simulink model "dbe_xaui_corr"  (Simulink 7.0)
settings: Solver=ode45  StartTime=0.0  StopTime=1000  RelTol=1e-3
undefined symbols (not defined in the file or in its folder): iBOB
libraries: xbsIndex_r4 x458, xps_library x38, casper_library_misc x12, casper_library_sources x2, gavrt_library x1, simulink x1, casper_library_scopes x1
(part 2 of 4)

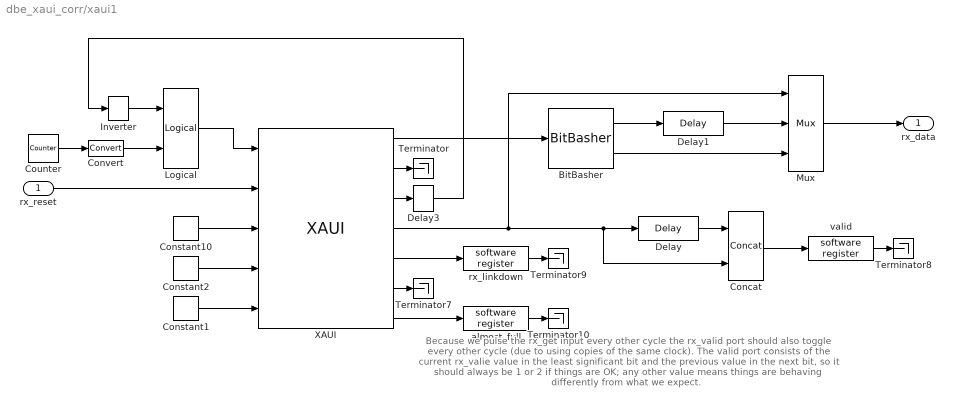
== system dbe_xaui_corr/xaui1 ==
  note: Because we pulse the rx_get input every other cycle
      | the rx_valid port should also toggle every other cycle
      | (due to using copies of the same clock).  The valid port
      | consists of the current rx_valie value in the least significant
      | bit and the previous value in the next bit, so it should
      | always be 1 or 2 if things are OK; any other value means
      | things are behaving differently from what we expect.
  rx_reset : Inport
  BitBasher : xbsIndex_r4/BitBasher  bitexpr=|  display_expr=off  sr_1=1  arith_type1=Unsigned  bin_pt1=0  sr_2=2  arith_type2=Unsigned  bin_pt2=0  sr_3=3  arith_type3=Unsigned  bin_pt3=0  sr_4=4  arith_type4=Unsigned  bin_pt4=0  dbl_ovrd=off  block_type=bitbasher
      | <html><head><meta name="qrichtext" content="1" /><style type="text/css">
      | p, li { white-space: pre-wrap; }
      | </style></head><body style=" font-family:'MS Shell Dlg 2'; font-size:8.25pt; font-weight:400; font-style:normal;">
      | <p style=" margin-top:12px; margin-bottom:12px; margin-left:0px; margin-right:0px; -qt-block-indent:0; text-indent:0px; font-family:'MS Shell Dlg'; font-size:8pt;">lo32={in64[31:0]}<br />hi32={in64[63:32]}</p></body></html>
      settings: block_version=10.1.3
  Concat : xbsIndex_r4/Concat  num_inputs=2  dbl_ovrd=off  block_type=concat
      settings: block_version=10.1.3
  Constant1 : xbsIndex_r4/Constant  arith_type=Boolean  const=0  n_bits=4  bin_pt=0  explicit_period=on  period=1  equ=P=C  opselect=C  inp2=PCIN>>17  opr=+  inp1=P  carry=CIN  dbl_ovrd=off  block_type=constant
      settings: block_version=11.3
  Constant10 : xbsIndex_r4/Constant  arith_type=Unsigned  const=2^4 -1  n_bits=32  bin_pt=0  explicit_period=on  period=1  equ=P=C  opselect=C  inp2=PCIN>>17  opr=+  inp1=P  carry=CIN  dbl_ovrd=off  block_type=constant
      settings: block_version=11.3
  Constant2 : xbsIndex_r4/Constant  arith_type=Unsigned  const=0  n_bits=4  bin_pt=0  explicit_period=on  period=1  equ=P=C  opselect=C  inp2=PCIN>>17  opr=+  inp1=P  carry=CIN  dbl_ovrd=off  block_type=constant
      settings: block_version=11.3
  Convert : xbsIndex_r4/Convert  arith_type=Boolean  n_bits=16  bin_pt=14  quantization=Truncate  overflow=Wrap  latency=0  dbl_ovrd=off  pipeline=off  block_type=convert
      settings: block_version=10.1.3
  Counter : xbsIndex_r4/Counter  cnt_type=Free Running  cnt_to=Inf  operation=Up  start_count=0  cnt_by_val=1  arith_type=Unsigned  n_bits=1  bin_pt=0  load_pin=off  rst=off  en=off  explicit_period=on  period=1  dbl_ovrd=off  use_behavioral_HDL=off  use_rpm=off  implementation=Fabric  block_type=counter
  Delay : xbsIndex_r4/Delay  en=off  latency=1  dbl_ovrd=off  reg_retiming=off  block_type=delay
  Delay1 : xbsIndex_r4/Delay  en=off  latency=1  dbl_ovrd=off  reg_retiming=off  block_type=delay
  Delay3 : xbsIndex_r4/Delay  en=off  latency=32  dbl_ovrd=off  reg_retiming=off  block_type=delay
      settings: block_version=11.3
  Inverter : xbsIndex_r4/Inverter  en=off  latency=0  dbl_ovrd=off  block_type=inv
      settings: block_version=11.3
  Logical : xbsIndex_r4/Logical  logical_function=AND  inputs=2  en=off  latency=0  precision=Full  arith_type=Unsigned  n_bits=16  bin_pt=0  align_bp=on  dbl_ovrd=off  block_type=logical
  Mux : xbsIndex_r4/Mux  inputs=2  en=off  latency=0  precision=Full  arith_type=Unsigned  n_bits=16  bin_pt=14  quantization=Truncate  overflow=Wrap  dbl_ovrd=off  block_type=mux
  Terminator{,7..10} (5 alike) : Terminator
  XAUI : xps_library/XAUI  Tag=xps:xaui  SystemSampleTime=-1  demux=1  port=iBOB:0  open_phy=off  show_param=off  pre_emph=3  swing=800
      link override convert_tx_data: n_bits=32
      link override convert_tx_outofband: n_bits=4
      link override dbe_xaui_corr_xaui1_XAUI_rx_data: n_bits=64
      link override dbe_xaui_corr_xaui1_XAUI_rx_outofband: n_bits=8
      link override dbe_xaui_corr_xaui_summer_XAUI0_rx_data: n_bits=32
      link override dbe_xaui_corr_xaui_summer_XAUI0_rx_outofband: n_bits=4
      link override dbe_xaui_xaui_summer_XAUI0_rx_data: n_bits=32
      link override dbe_xaui_xaui_summer_XAUI0_rx_outofband: n_bits=4
      link override xaui_XAUI_RECV_rx_data: n_bits=32
      link override xaui_XAUI_RECV_rx_outofband: n_bits=4
  almost_full : xps_library/software register  Tag=xps:sw_reg  SystemSampleTime=-1  io_dir=To Processor  arith_type=Unsigned  bitwidth=32  bin_pt=0  sample_period=1  gw_name=dbe_xaui_corr_xaui1_almost_full_user_data_in
      link override convert: arith_type=Unsigned  n_bits=32  bin_pt=0
  rx_linkdown : xps_library/software register  Tag=xps:sw_reg  SystemSampleTime=-1  io_dir=To Processor  arith_type=Unsigned  bitwidth=32  bin_pt=0  sample_period=1  gw_name=dbe_xaui_corr_xaui1_rx_linkdown_user_data_in
      link override convert: arith_type=Unsigned  n_bits=32  bin_pt=0
  valid : xps_library/software register  Tag=xps:sw_reg  SystemSampleTime=-1  io_dir=To Processor  arith_type=Unsigned  bitwidth=32  bin_pt=0  sample_period=1  gw_name=dbe_xaui_corr_xaui1_valid_user_data_in
      link override convert: arith_type=Unsigned  n_bits=32  bin_pt=0
  rx_data : Outport
  wires:
  XAUI/2 -> Terminator/1
  Constant2/1 -> XAUI/4
  XAUI/3 -> Delay3/1
  Delay3/1 -> Inverter/1
  XAUI/6 -> Terminator7/1
  Constant10/1 -> XAUI/3
  XAUI/4 -> Mux/1, Delay/1, Concat/2
  XAUI/5 -> rx_linkdown/1
  valid/1 -> Terminator8/1
  rx_linkdown/1 -> Terminator9/1
  almost_full/1 -> Terminator10/1
  XAUI/7 -> almost_full/1
  Constant1/1 -> XAUI/5
  rx_reset/1 -> XAUI/2
  Inverter/1 -> Logical/1
  Logical/1 -> XAUI/1
  Counter/1 -> Convert/1
  BitBasher/2 -> Mux/3
  BitBasher/1 -> Delay1/1
  Delay1/1 -> Mux/2
  XAUI/1 -> BitBasher/1
  Mux/1 -> rx_data/1
  Concat/1 -> valid/1
  Delay/1 -> Concat/1
  Convert/1 -> Logical/2

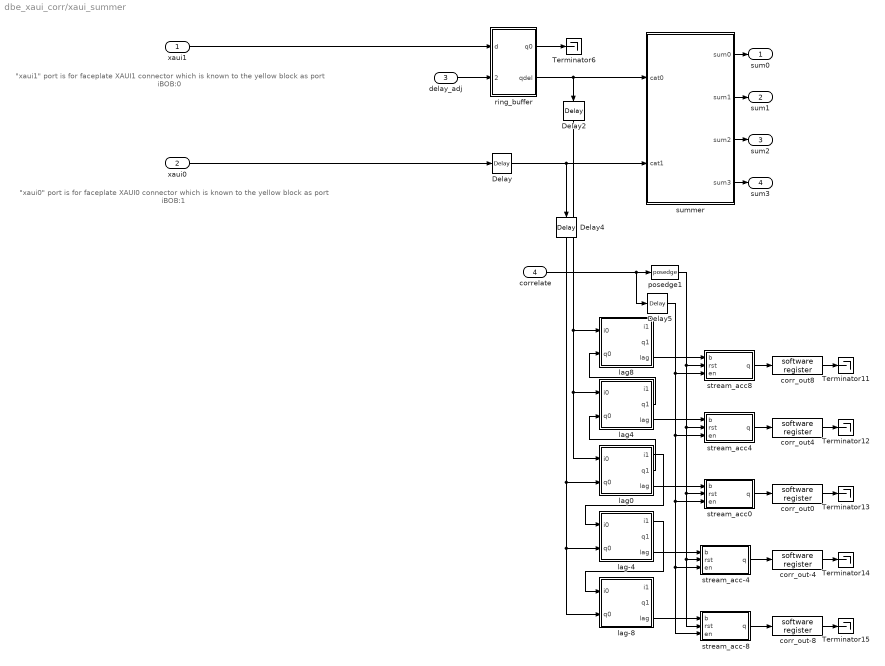
== system dbe_xaui_corr/xaui_summer ==
  note: "xaui1" port is for faceplate XAUI1 connector
      | which is known to the yellow block as port iBOB:0
  note: "xaui0" port is for faceplate XAUI0 connector
      | which is known to the yellow block as port iBOB:1
  xaui1 : Inport  OutDataType=sfix(16)  OutScaling=2^0
  xaui0 : Inport  Port=2  OutDataType=sfix(16)  OutScaling=2^0
  delay_adj : Inport  Port=3  OutDataType=sfix(16)  OutScaling=2^0
  correlate : Inport  Port=4  OutDataType=sfix(16)  OutScaling=2^0
  Delay : xbsIndex_r4/Delay  en=off  latency=8  dbl_ovrd=off  reg_retiming=on  block_type=delay
  Delay2 : xbsIndex_r4/Delay  Orientation=down  en=off  latency=8  dbl_ovrd=off  reg_retiming=on  block_type=delay
  Delay4 : xbsIndex_r4/Delay  Orientation=down  en=off  latency=8  dbl_ovrd=off  reg_retiming=on  block_type=delay
  Delay5 : xbsIndex_r4/Delay  en=off  latency=2  dbl_ovrd=off  reg_retiming=on  block_type=delay
  Terminator{6,11..15} (6 alike) : Terminator
  corr_out-4 : xps_library/software register  Tag=xps:sw_reg  SystemSampleTime=-1  io_dir=To Processor  arith_type="Signed  (2's comp)"  bitwidth=32  bin_pt=14  sample_period=1  gw_name=dbe_xaui_corr_xaui_summer_corr_out_4_user_data_in
      link override convert: arith_type="Signed  (2's comp)"  n_bits=32  bin_pt=14
  corr_out-8 : xps_library/software register  Tag=xps:sw_reg  SystemSampleTime=-1  io_dir=To Processor  arith_type="Signed  (2's comp)"  bitwidth=32  bin_pt=14  sample_period=1  gw_name=dbe_xaui_corr_xaui_summer_corr_out_8_user_data_in
      link override convert: arith_type="Signed  (2's comp)"  n_bits=32  bin_pt=14
  corr_out0 : xps_library/software register  Tag=xps:sw_reg  SystemSampleTime=-1  io_dir=To Processor  arith_type="Signed  (2's comp)"  bitwidth=32  bin_pt=14  sample_period=1  gw_name=dbe_xaui_corr_xaui_summer_corr_out0_user_data_in
      link override convert: arith_type="Signed  (2's comp)"  n_bits=32  bin_pt=14
  corr_out4 : xps_library/software register  Tag=xps:sw_reg  SystemSampleTime=-1  io_dir=To Processor  arith_type="Signed  (2's comp)"  bitwidth=32  bin_pt=14  sample_period=1  gw_name=dbe_xaui_corr_xaui_summer_corr_out4_user_data_in
      link override convert: arith_type="Signed  (2's comp)"  n_bits=32  bin_pt=14
  corr_out8 : xps_library/software register  Tag=xps:sw_reg  SystemSampleTime=-1  io_dir=To Processor  arith_type="Signed  (2's comp)"  bitwidth=32  bin_pt=14  sample_period=1  gw_name=dbe_xaui_corr_xaui_summer_corr_out8_user_data_in
      link override convert: arith_type="Signed  (2's comp)"  n_bits=32  bin_pt=14
  lag-4 : Subsystem
  lag-8 : Subsystem
  lag0 : Subsystem
  lag4 : Subsystem
  lag8 : Subsystem
  posedge1 : casper_library_misc/posedge  Tag=Rising Edge Detector  SystemSampleTime=-1
  ring_buffer : Subsystem
  stream_acc-4 : Subsystem  mask{data_type=Signed, bits=32, bin_pt=14, add_latency=4}
      mask prompts: data_type "Output Data Type"; bits "Output Bit Width:"; bin_pt "Output Binary Point:"; add_latency "Adder Latency"
      mask StyleString: popup(Signed|Unsigned),edit,edit,edit
  stream_acc-8 : Subsystem  mask{data_type=Signed, bits=32, bin_pt=14, add_latency=4}
      mask prompts: data_type "Output Data Type"; bits "Output Bit Width:"; bin_pt "Output Binary Point:"; add_latency "Adder Latency"
      mask StyleString: popup(Signed|Unsigned),edit,edit,edit
  stream_acc0 : Subsystem  mask{data_type=Signed, bits=32, bin_pt=14, add_latency=4}
      mask prompts: data_type "Output Data Type"; bits "Output Bit Width:"; bin_pt "Output Binary Point:"; add_latency "Adder Latency"
      mask StyleString: popup(Signed|Unsigned),edit,edit,edit
  stream_acc4 : Subsystem  mask{data_type=Signed, bits=32, bin_pt=14, add_latency=4}
      mask prompts: data_type "Output Data Type"; bits "Output Bit Width:"; bin_pt "Output Binary Point:"; add_latency "Adder Latency"
      mask StyleString: popup(Signed|Unsigned),edit,edit,edit
  stream_acc8 : Subsystem  mask{data_type=Signed, bits=32, bin_pt=14, add_latency=4}
      mask prompts: data_type "Output Data Type"; bits "Output Bit Width:"; bin_pt "Output Binary Point:"; add_latency "Adder Latency"
      mask StyleString: popup(Signed|Unsigned),edit,edit,edit
  summer : Subsystem
  sum0 : Outport
  sum1 : Outport  Port=2
  sum2 : Outport  Port=3
  sum3 : Outport  Port=4
  wires:
  summer/1(sum0) -> sum0/1
  summer/2(sum1) -> sum1/1
  summer/3(sum2) -> sum2/1
  summer/4(sum3) -> sum3/1
  xaui1/1 -> ring_buffer/1(d)
  Delay/1 -> summer/2(cat1), Delay4/1
  ring_buffer/2(qdel) -> summer/1(cat0), Delay2/1
  ring_buffer/1(q0) -> Terminator6/1
  lag0/2(q1) -> lag4/2(q0)
  lag4/2(q1) -> lag8/2(q0)
  lag0/1(i1) -> lag-4/1(i0)
  lag-4/1(i1) -> lag-8/1(i0)
  lag8/3(lag) -> stream_acc8/1(b)
  lag4/3(lag) -> stream_acc4/1(b)
  lag0/3(lag) -> stream_acc0/1(b)
  lag-8/3(lag) -> stream_acc-8/1(b)
  correlate/1 -> Delay5/1, posedge1/1
  Delay5/1 -> stream_acc-4/3(en), stream_acc-8/3(en), stream_acc0/3(en), stream_acc4/3(en), stream_acc8/3(en)
  posedge1/1 -> stream_acc-4/2(rst), stream_acc-8/2(rst), stream_acc0/2(rst), stream_acc4/2(rst), stream_acc8/2(rst)
  delay_adj/1 -> ring_buffer/2(delay)
  corr_out8/1 -> Terminator11/1
  stream_acc8/1(q) -> corr_out8/1
  corr_out4/1 -> Terminator12/1
  stream_acc4/1(q) -> corr_out4/1
  corr_out0/1 -> Terminator13/1
  stream_acc0/1(q) -> corr_out0/1
  corr_out-4/1 -> Terminator14/1
  stream_acc-4/1(q) -> corr_out-4/1
  corr_out-8/1 -> Terminator15/1
  stream_acc-8/1(q) -> corr_out-8/1
  lag-4/3(lag) -> stream_acc-4/1(b)
  Delay2/1 -> lag4/1(i0), lag0/1(i0), lag8/1(i0)
  Delay4/1 -> lag-4/2(q0), lag-8/2(q0), lag0/2(q0)
  xaui0/1 -> Delay/1

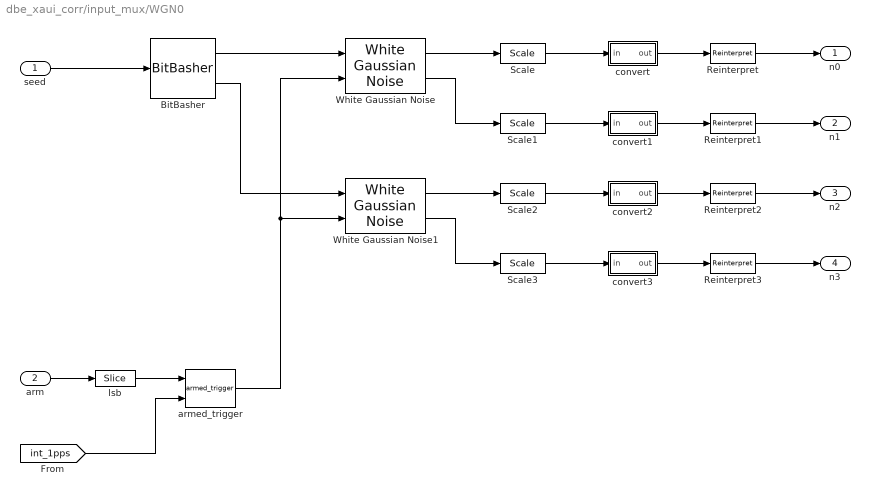
== system dbe_xaui_corr/input_mux/WGN0 ==
  seed : Inport
  arm : Inport  Port=2
  BitBasher : xbsIndex_r4/BitBasher  bitexpr=|  display_expr=off  sr_1=1  arith_type1=Unsigned  bin_pt1=0  sr_2=2  arith_type2=Unsigned  bin_pt2=0  sr_3=3  arith_type3=Unsigned  bin_pt3=0  sr_4=4  arith_type4=Unsigned  bin_pt4=0  dbl_ovrd=off  block_type=bitbasher
      | <html><head><meta name="qrichtext" content="1" /><style type="text/css">
      | p, li { white-space: pre-wrap; }
      | </style></head><body style=" font-family:'MS Shell Dlg 2'; font-size:8.25pt; font-weight:400; font-style:normal;">
      | <p style=" margin-top:12px; margin-bottom:12px; margin-left:0px; margin-right:0px; -qt-block-indent:0; text-indent:0px; font-family:'MS Shell Dlg'; font-size:8pt;">s0={8'h55,s[15:0],8'haa}<br />s1={8'h55,s[31:16],8'haa}</p></body></html>
      settings: block_version=10.1.3
  Reinterpret{,1..3} (4 alike) : xbsIndex_r4/Reinterpret  force_arith_type=off  arith_type=Unsigned  force_bin_pt=on  bin_pt=7  block_type=reinterpret
      settings: infoedit="Changes signal type without altering the binary representation.   You can changed the signal between signed and unsigned, and relocate the binary point.<P><P>Hardware notes: In hardware this block costs nothing.<P><P>Example:  Suppose the input is 6 bits wide, signed, with 2 fractional bits, and the output is forced to unsigned with 0 fractional bits.  Then an input of -2.0 (1110.00 in binary 2's complement) becomes an output of 56 (111000 in binary)."  block_version=10.1.3
  Scale{,1..3} (4 alike) : xbsIndex_r4/Scale  scale_factor=4  dbl_ovrd=off  block_type=scale
      settings: infoedit=Scales input by a power of two by adjusting the binary point position.<P><P>Hardware notes: In hardware this block costs nothing.  block_version=10.1.3
  White Gaussian Noise : casper_library_sources/White Gaussian Noise  SystemSampleTime=-1  seed=hex2dec('55ffffaa')
      link override tt800_uprng/tt800_seed_gen/LFSR: rst_value='12345678'
  White Gaussian Noise1 : casper_library_sources/White Gaussian Noise  SystemSampleTime=-1  seed=hex2dec('550000aa')
      link override tt800_uprng/tt800_seed_gen/LFSR: rst_value='12345678'
  armed_trigger : casper_library_misc/armed_trigger  SystemSampleTime=-1  hidden=0
  convert : Subsystem  AncestorBlock=casper_library/Misc/convert  mask(convert){bin_pt_in=10, n_bits_out=8, bin_pt_out=0, quantization=Round  (unbiased: +/- Inf), overflow=Wrap, latency=1}
      mask prompts: bin_pt_in "Binary Point In"; n_bits_out "Bit Width Out"; bin_pt_out "Binary Point Out"
      mask help:
      | Convert input value to the specified bit width and precision.
      |
      | Does not support upscaling number of fractional bits (eg 8_5 to 8_4 is ok, but not 8_4 to 8_5).
      mask init:
      | convert_init(gcb, ...
      |     'bin_pt_in',bin_pt_in, ...
      |     'n_bits_out',n_bits_out,...
      |     'bin_pt_out',bin_pt_out, ...
      |     'quantization',quantization,...
      |     'overflow',overflow,...
      |     'latency',latency);
      settings: AttributesFormatString=|
      | N_10 ==> 8_0
      | round inf, wrap
      | latency = 1
      mask Help:
      | <pre>
      | Description::
      | 
      | Outputs converted version of the input.
      | 
      | Mask Parameters::
      | 
      | Binary Point In (bin_pt_in): Specifies the binary point location in the input.
      | 
      | Bit Width Out (n_bits_out): Specifies the width of the output.
      | 
      | Binary Point Out (bin_pt_out): Specifies the binary point location in the output.
      | 
      | Quantization (quantization): Specifies quantization handling.
      | 
      | Overflow (overflow): Specifies overflow handling.
      | 
      | Latency (latency): Specifies the latency of the underlying adder block, which is the overall
      | latency of this block as well.
      | </pre>
      mask StyleString: edit,edit,edit,popup(Truncate|Round  (unbiased: +/- Inf)|Round  (unbiased: Even Values)|Round  (unbiased: Zero)|Round  (unbiased: Odd Values)|Round  (biased: Up)|Round  (biased: Down)),popup(Wrap|Saturate|Error),edit
  convert1 : Subsystem  AncestorBlock=casper_library/Misc/convert  mask(convert){bin_pt_in=10, n_bits_out=8, bin_pt_out=0, quantization=Round  (unbiased: +/- Inf), overflow=Wrap, latency=1}
      mask prompts: bin_pt_in "Binary Point In"; n_bits_out "Bit Width Out"; bin_pt_out "Binary Point Out"
      mask help:
      | Convert input value to the specified bit width and precision.
      |
      | Does not support upscaling number of fractional bits (eg 8_5 to 8_4 is ok, but not 8_4 to 8_5).
      mask init: same as dbe_xaui_corr/input_mux/WGN0/convert
      settings: AttributesFormatString=|
      | N_10 ==> 8_0
      | round inf, wrap
      | latency = 1
      mask Help:
      | <pre>
      | Description::
      | 
      | Outputs converted version of the input.
      | 
      | Mask Parameters::
      | 
      | Binary Point In (bin_pt_in): Specifies the binary point location in the input.
      | 
      | Bit Width Out (n_bits_out): Specifies the width of the output.
      | 
      | Binary Point Out (bin_pt_out): Specifies the binary point location in the output.
      | 
      | Quantization (quantization): Specifies quantization handling.
      | 
      | Overflow (overflow): Specifies overflow handling.
      | 
      | Latency (latency): Specifies the latency of the underlying adder block, which is the overall
      | latency of this block as well.
      | </pre>
      mask StyleString: edit,edit,edit,popup(Truncate|Round  (unbiased: +/- Inf)|Round  (unbiased: Even Values)|Round  (unbiased: Zero)|Round  (unbiased: Odd Values)|Round  (biased: Up)|Round  (biased: Down)),popup(Wrap|Saturate|Error),edit
  convert2 : Subsystem  AncestorBlock=casper_library/Misc/convert  mask(convert){bin_pt_in=10, n_bits_out=8, bin_pt_out=0, quantization=Round  (unbiased: +/- Inf), overflow=Wrap, latency=1}
      mask prompts: bin_pt_in "Binary Point In"; n_bits_out "Bit Width Out"; bin_pt_out "Binary Point Out"
      mask help:
      | Convert input value to the specified bit width and precision.
      |
      | Does not support upscaling number of fractional bits (eg 8_5 to 8_4 is ok, but not 8_4 to 8_5).
      mask init: same as dbe_xaui_corr/input_mux/WGN0/convert
      settings: AttributesFormatString=|
      | N_10 ==> 8_0
      | round inf, wrap
      | latency = 1
      mask Help:
      | <pre>
      | Description::
      | 
      | Outputs converted version of the input.
      | 
      | Mask Parameters::
      | 
      | Binary Point In (bin_pt_in): Specifies the binary point location in the input.
      | 
      | Bit Width Out (n_bits_out): Specifies the width of the output.
      | 
      | Binary Point Out (bin_pt_out): Specifies the binary point location in the output.
      | 
      | Quantization (quantization): Specifies quantization handling.
      | 
      | Overflow (overflow): Specifies overflow handling.
      | 
      | Latency (latency): Specifies the latency of the underlying adder block, which is the overall
      | latency of this block as well.
      | </pre>
      mask StyleString: edit,edit,edit,popup(Truncate|Round  (unbiased: +/- Inf)|Round  (unbiased: Even Values)|Round  (unbiased: Zero)|Round  (unbiased: Odd Values)|Round  (biased: Up)|Round  (biased: Down)),popup(Wrap|Saturate|Error),edit
  convert3 : Subsystem  AncestorBlock=casper_library/Misc/convert  mask(convert){bin_pt_in=10, n_bits_out=8, bin_pt_out=0, quantization=Round  (unbiased: +/- Inf), overflow=Wrap, latency=1}
      mask prompts: bin_pt_in "Binary Point In"; n_bits_out "Bit Width Out"; bin_pt_out "Binary Point Out"
      mask help:
      | Convert input value to the specified bit width and precision.
      |
      | Does not support upscaling number of fractional bits (eg 8_5 to 8_4 is ok, but not 8_4 to 8_5).
      mask init: same as dbe_xaui_corr/input_mux/WGN0/convert
      settings: AttributesFormatString=|
      | N_10 ==> 8_0
      | round inf, wrap
      | latency = 1
      mask Help:
      | <pre>
      | Description::
      | 
      | Outputs converted version of the input.
      | 
      | Mask Parameters::
      | 
      | Binary Point In (bin_pt_in): Specifies the binary point location in the input.
      | 
      | Bit Width Out (n_bits_out): Specifies the width of the output.
      | 
      | Binary Point Out (bin_pt_out): Specifies the binary point location in the output.
      | 
      | Quantization (quantization): Specifies quantization handling.
      | 
      | Overflow (overflow): Specifies overflow handling.
      | 
      | Latency (latency): Specifies the latency of the underlying adder block, which is the overall
      | latency of this block as well.
      | </pre>
      mask StyleString: edit,edit,edit,popup(Truncate|Round  (unbiased: +/- Inf)|Round  (unbiased: Even Values)|Round  (unbiased: Zero)|Round  (unbiased: Odd Values)|Round  (biased: Up)|Round  (biased: Down)),popup(Wrap|Saturate|Error),edit
  lsb : xbsIndex_r4/Slice  nbits=1  boolean_output=on  mode=Lower Bit Location + Width  bit1=0  base1=MSB of Input  bit0=0  base0=LSB of Input  dbl_ovrd=off  block_type=slice
      settings: infoedit="Extracts a given range of bits from each input sample and presents it at the output.  The output type is ordinarily unsigned with binary point at zero, but can be Boolean when the slice is one bit wide.<P><P>Hardware notes: In hardware this block costs nothing."  block_version=10.1.3
  n0 : Outport
  n1 : Outport  Port=2
  n2 : Outport  Port=3
  n3 : Outport  Port=4
  wires:
  convert/1(out) -> Reinterpret/1
  Scale/1 -> convert/1(in)
  convert1/1(out) -> Reinterpret1/1
  Scale1/1 -> convert1/1(in)
  White Gaussian Noise/1 -> Scale/1
  White Gaussian Noise/2 -> Scale1/1
  Reinterpret/1 -> n0/1
  Reinterpret1/1 -> n1/1
  armed_trigger/1 -> White Gaussian Noise/2, White Gaussian Noise1/2
  arm/1 -> lsb/1
  [int_1pps] -> armed_trigger/2
  convert2/1(out) -> Reinterpret2/1
  Scale2/1 -> convert2/1(in)
  convert3/1(out) -> Reinterpret3/1
  Scale3/1 -> convert3/1(in)
  White Gaussian Noise1/1 -> Scale2/1
  White Gaussian Noise1/2 -> Scale3/1
  Reinterpret2/1 -> n2/1
  Reinterpret3/1 -> n3/1
  BitBasher/1 -> White Gaussian Noise/1
  seed/1 -> BitBasher/1
  BitBasher/2 -> White Gaussian Noise1/1
  lsb/1 -> armed_trigger/1

== system dbe_xaui_corr/onepps_sync/armshake ==
  ext_1pps : Inport  OutDataType=sfix(16)  OutScaling=2^0
  ext_arm1pps : Inport  Port=2  OutDataType=sfix(16)  OutScaling=2^0
  Constant : xbsIndex_r4/Constant  arith_type=Unsigned  const=1  n_bits=1  bin_pt=0  explicit_period=on  period=1  equ=P=C  opselect=C  inp2=PCIN>>17  opr=+  inp1=P  carry=CIN  dbl_ovrd=off  block_type=constant
      settings: block_version=11.3
  Constant1 : xbsIndex_r4/Constant  arith_type=Unsigned  const=1  n_bits=1  bin_pt=0  explicit_period=on  period=1  equ=P=C  opselect=C  inp2=PCIN>>17  opr=+  inp1=P  carry=CIN  dbl_ovrd=off  block_type=constant
      settings: block_version=11.3
  Convert : xbsIndex_r4/Convert  arith_type=Boolean  n_bits=8  bin_pt=6  quantization=Truncate  overflow=Wrap  latency=0  dbl_ovrd=off  pipeline=off  block_type=convert
      settings: xl_area=[0, 0, 0, 0, 0, 0, 0]  block_version=11.3
  Convert1 : xbsIndex_r4/Convert  arith_type=Boolean  n_bits=8  bin_pt=6  quantization=Truncate  overflow=Wrap  latency=0  dbl_ovrd=off  pipeline=off  block_type=convert
      settings: xl_area=[0, 0, 0, 0, 0, 0, 0]  block_version=11.3
  Convert2 : xbsIndex_r4/Convert  arith_type=Boolean  n_bits=8  bin_pt=6  quantization=Truncate  overflow=Wrap  latency=0  dbl_ovrd=off  pipeline=off  block_type=convert
      settings: xl_area=[0, 0, 0, 0, 0, 0, 0]  block_version=11.3
  Expression : xbsIndex_r4/Expression  expression=a & ~b  align_bp=on  en=off  latency=0  precision=Full  arith_type=Unsigned  n_bits=8  bin_pt=2  dbl_ovrd=off  block_type=expr
      settings: xl_area=[0, 0, 0, 0, 0, 0, 0]  block_version=11.3
  Expression1 : xbsIndex_r4/Expression  expression=~a & b  align_bp=on  en=off  latency=0  precision=Full  arith_type=Unsigned  n_bits=8  bin_pt=2  dbl_ovrd=off  block_type=expr
      settings: xl_area=[0, 0, 0, 0, 0, 0, 0]  block_version=11.3
  Expression2 : xbsIndex_r4/Expression  expression=(a & ~b) & c  align_bp=on  en=off  latency=1  precision=Full  arith_type=Unsigned  n_bits=8  bin_pt=2  dbl_ovrd=off  block_type=expr
      settings: xl_area=[0, 0, 0, 0, 0, 0, 0]  block_version=11.3
  Register : xbsIndex_r4/Register  init=0  rst=off  en=off  dbl_ovrd=off  block_type=register
      settings: xl_area=[0, 0, 0, 0, 0, 0, 0]  block_version=11.3
  Register1 : xbsIndex_r4/Register  init=0  rst=on  en=on  dbl_ovrd=off  block_type=register
      settings: xl_area=[0, 0, 0, 0, 0, 0, 0]  block_version=11.3
  Register2 : xbsIndex_r4/Register  init=0  rst=on  en=on  dbl_ovrd=off  block_type=register
      settings: xl_area=[0, 0, 0, 0, 0, 0, 0]  block_version=11.3
  Register3 : xbsIndex_r4/Register  init=0  rst=off  en=off  dbl_ovrd=off  block_type=register
      settings: xl_area=[0, 0, 0, 0, 0, 0, 0]  block_version=11.3
  Slice8 : xbsIndex_r4/Slice  nbits=1  boolean_output=off  mode=Lower Bit Location + Width  bit1=0  base1=MSB of Input  bit0=0  base0=LSB of Input  dbl_ovrd=off  block_type=slice
      settings: block_version=11.3
  rst_1pps : Outport  OutDataType=sfix(16)  OutScaling=2^0
  arm_ack : Outport  Port=2  OutDataType=sfix(16)  OutScaling=2^0
  wires:
  Register/1 -> Expression/2, Expression1/2
  Convert/1 -> Expression2/3
  Register3/1 -> Expression2/2
  Slice8/1 -> Expression/1, Register/1, Expression1/1
  Register1/1 -> Convert/1
  ext_1pps/1 -> Expression2/1, Register3/1
  Expression2/1 -> rst_1pps/1, Register1/2, Register2/3
  ext_arm1pps/1 -> Slice8/1
  Constant/1 -> Register1/1
  Expression/1 -> Convert1/1
  Constant1/1 -> Register2/1
  Expression1/1 -> Convert2/1
  Register2/1 -> arm_ack/1
  Convert1/1 -> Register1/3
  Convert2/1 -> Register2/2

== system dbe_xaui_corr/onepps_sync/int_1pps_gen ==
  rst : Inport  OutDataType=sfix(16)  OutScaling=2^0
  1pps_gen : Subsystem
  Simulation Multiplexer : xbsIndex_r4/Simulation Multiplexer  sim_sel=2  hw_sel=1  block_type=simmux
      settings: infoedit="Distinguish input subsystems as \"simulation only\" and \"generation only\".  The input specified For Simulation will be used during Simulink simulation.  The input specified For Generation will be used during code generation.  This block will typically be used on the output of a HW Co-Simulation, Black Box, or ModelSim subsystem.<br><br>Hardware Notes: This block costs nothing."  block_version=11.3
  sim1pps_gen : Subsystem
  1pps : Outport  OutDataType=sfix(16)  OutScaling=2^0
  wires:
  Simulation Multiplexer/1 -> 1pps/1
  rst/1 -> sim1pps_gen/1(rst), 1pps_gen/1(rst)
  sim1pps_gen/1(1pps_sim) -> Simulation Multiplexer/2
  1pps_gen/1(1pps) -> Simulation Multiplexer/1

== system dbe_xaui_corr/xaui_summer/lag-4 ==
  i0 : Inport  OutDataType=sfix(16)  OutScaling=2^0
  q0 : Inport  Port=2  OutDataType=sfix(16)  OutScaling=2^0
  AddSub : xbsIndex_r4/AddSub  mode=Addition  use_carryin=off  use_carryout=off  en=off  latency=2  precision=Full  arith_type=Unsigned  n_bits=16  bin_pt=14  quantization=Truncate  overflow=Wrap  dbl_ovrd=off  use_behavioral_HDL=off  pipelined=off  use_rpm=on  hw_selection=Fabric  block_type=addsub
      settings: block_version=10.1.3
  AddSub1 : xbsIndex_r4/AddSub  mode=Addition  use_carryin=off  use_carryout=off  en=off  latency=2  precision=Full  arith_type=Unsigned  n_bits=16  bin_pt=14  quantization=Truncate  overflow=Wrap  dbl_ovrd=off  use_behavioral_HDL=off  pipelined=off  use_rpm=on  hw_selection=Fabric  block_type=addsub
      settings: block_version=10.1.3
  AddSub2 : xbsIndex_r4/AddSub  mode=Addition  use_carryin=off  use_carryout=off  en=off  latency=2  precision=Full  arith_type=Unsigned  n_bits=16  bin_pt=14  quantization=Truncate  overflow=Wrap  dbl_ovrd=off  use_behavioral_HDL=off  pipelined=off  use_rpm=on  hw_selection=Fabric  block_type=addsub
      settings: block_version=10.1.3
  Delay : xbsIndex_r4/Delay  en=off  latency=1  dbl_ovrd=off  reg_retiming=off  block_type=delay
  Delay1 : xbsIndex_r4/Delay  en=off  latency=1  dbl_ovrd=off  reg_retiming=off  block_type=delay
  Mult{,1..3} (4 alike) : xbsIndex_r4/Mult  precision=Full  arith_type="Signed  (2's comp)"  n_bits=16  bin_pt=14  quantization=Truncate  overflow=Wrap  en=off  latency=5  dbl_ovrd=off  use_behavioral_HDL=on  use_embedded=off  opt=Speed  optimum_pipeline=on  pipeline=on  use_rpm=on  placement_style=Triangular  block_type=mult
      settings: infoedit=Hardware notes: To use the internal pipeline stage of the dedicated multiplier you must select 'Pipeline for maximum performance'.  block_version=10.1.3
  uncram : Subsystem  AncestorBlock=gavrt_library/uncram  mask(uncram){num_slice=4, slice_width=8, bin_pt=7, arith_type=1}
      mask prompts: num_slice "Number of slices"; slice_width "Slice Width"; bin_pt "Output Binary Point"; arith_type "Output Arithmetic Type (0=Unsigned, 1=Signed)"
      mask help: Takes a concatenated input and slices it up into even pieces and reinterprets them as signed fixed point numbers with a given binary point.
      mask init:
      | uncram_init(gcb, ...
      |     'num_slice', num_slice, ...
      |     'slice_width', slice_width, ...
      |     'bin_pt', bin_pt, ...
      |     'arith_type', arith_type);
      settings: AttributesFormatString=Fix_8_7
  uncram1 : Subsystem  AncestorBlock=gavrt_library/uncram  mask(uncram){num_slice=4, slice_width=8, bin_pt=7, arith_type=1}
      mask prompts: num_slice "Number of slices"; slice_width "Slice Width"; bin_pt "Output Binary Point"; arith_type "Output Arithmetic Type (0=Unsigned, 1=Signed)"
      mask help: Takes a concatenated input and slices it up into even pieces and reinterprets them as signed fixed point numbers with a given binary point.
      mask init:
      | uncram_init(gcb, ...
      |     'num_slice', num_slice, ...
      |     'slice_width', slice_width, ...
      |     'bin_pt', bin_pt, ...
      |     'arith_type', arith_type);
      settings: AttributesFormatString=Fix_8_7
  i1 : Outport  OutDataType=sfix(16)  OutScaling=2^0
  q1 : Outport  Port=2  OutDataType=sfix(16)  OutScaling=2^0
  lag : Outport  Port=3  OutDataType=sfix(16)  OutScaling=2^0
  wires:
  AddSub2/1 -> lag/1
  AddSub1/1 -> AddSub2/2
  AddSub/1 -> AddSub2/1
  Mult3/1 -> AddSub1/2
  Mult2/1 -> AddSub1/1
  Mult1/1 -> AddSub/2
  Mult/1 -> AddSub/1
  uncram1/4(Out4) -> Mult3/2
  uncram1/3(Out3) -> Mult2/2
  uncram1/2(Out2) -> Mult1/2
  uncram1/1(Out1) -> Mult/2
  uncram/4(Out4) -> Mult3/1
  uncram/3(Out3) -> Mult2/1
  uncram/2(Out2) -> Mult1/1
  uncram/1(Out1) -> Mult/1
  Delay1/1 -> q1/1
  Delay/1 -> i1/1
  q0/1 -> Delay1/1, uncram1/1(In)
  i0/1 -> Delay/1, uncram/1(In)

== system dbe_xaui_corr/xaui_summer/lag-8 ==
  i0 : Inport  OutDataType=sfix(16)  OutScaling=2^0
  q0 : Inport  Port=2  OutDataType=sfix(16)  OutScaling=2^0
  AddSub : xbsIndex_r4/AddSub  mode=Addition  use_carryin=off  use_carryout=off  en=off  latency=2  precision=Full  arith_type=Unsigned  n_bits=16  bin_pt=14  quantization=Truncate  overflow=Wrap  dbl_ovrd=off  use_behavioral_HDL=off  pipelined=off  use_rpm=on  hw_selection=Fabric  block_type=addsub
      settings: block_version=10.1.3
  AddSub1 : xbsIndex_r4/AddSub  mode=Addition  use_carryin=off  use_carryout=off  en=off  latency=2  precision=Full  arith_type=Unsigned  n_bits=16  bin_pt=14  quantization=Truncate  overflow=Wrap  dbl_ovrd=off  use_behavioral_HDL=off  pipelined=off  use_rpm=on  hw_selection=Fabric  block_type=addsub
      settings: block_version=10.1.3
  AddSub2 : xbsIndex_r4/AddSub  mode=Addition  use_carryin=off  use_carryout=off  en=off  latency=2  precision=Full  arith_type=Unsigned  n_bits=16  bin_pt=14  quantization=Truncate  overflow=Wrap  dbl_ovrd=off  use_behavioral_HDL=off  pipelined=off  use_rpm=on  hw_selection=Fabric  block_type=addsub
      settings: block_version=10.1.3
  Delay : xbsIndex_r4/Delay  en=off  latency=1  dbl_ovrd=off  reg_retiming=off  block_type=delay
  Delay1 : xbsIndex_r4/Delay  en=off  latency=1  dbl_ovrd=off  reg_retiming=off  block_type=delay
  Mult{,1..3} (4 alike) : xbsIndex_r4/Mult  precision=Full  arith_type="Signed  (2's comp)"  n_bits=16  bin_pt=14  quantization=Truncate  overflow=Wrap  en=off  latency=5  dbl_ovrd=off  use_behavioral_HDL=on  use_embedded=off  opt=Speed  optimum_pipeline=on  pipeline=on  use_rpm=on  placement_style=Triangular  block_type=mult
      settings: infoedit=Hardware notes: To use the internal pipeline stage of the dedicated multiplier you must select 'Pipeline for maximum performance'.  block_version=10.1.3
  uncram : Subsystem  AncestorBlock=gavrt_library/uncram  mask(uncram){num_slice=4, slice_width=8, bin_pt=7, arith_type=1}
      mask prompts: num_slice "Number of slices"; slice_width "Slice Width"; bin_pt "Output Binary Point"; arith_type "Output Arithmetic Type (0=Unsigned, 1=Signed)"
      mask help: Takes a concatenated input and slices it up into even pieces and reinterprets them as signed fixed point numbers with a given binary point.
      mask init:
      | uncram_init(gcb, ...
      |     'num_slice', num_slice, ...
      |     'slice_width', slice_width, ...
      |     'bin_pt', bin_pt, ...
      |     'arith_type', arith_type);
      settings: AttributesFormatString=Fix_8_7
  uncram1 : Subsystem  AncestorBlock=gavrt_library/uncram  mask(uncram){num_slice=4, slice_width=8, bin_pt=7, arith_type=1}
      mask prompts: num_slice "Number of slices"; slice_width "Slice Width"; bin_pt "Output Binary Point"; arith_type "Output Arithmetic Type (0=Unsigned, 1=Signed)"
      mask help: Takes a concatenated input and slices it up into even pieces and reinterprets them as signed fixed point numbers with a given binary point.
      mask init:
      | uncram_init(gcb, ...
      |     'num_slice', num_slice, ...
      |     'slice_width', slice_width, ...
      |     'bin_pt', bin_pt, ...
      |     'arith_type', arith_type);
      settings: AttributesFormatString=Fix_8_7
  i1 : Outport  OutDataType=sfix(16)  OutScaling=2^0
  q1 : Outport  Port=2  OutDataType=sfix(16)  OutScaling=2^0
  lag : Outport  Port=3  OutDataType=sfix(16)  OutScaling=2^0
  wires:
  i0/1 -> uncram/1(In), Delay/1
  q0/1 -> uncram1/1(In), Delay1/1
  Delay/1 -> i1/1
  Delay1/1 -> q1/1
  uncram/1(Out1) -> Mult/1
  uncram/2(Out2) -> Mult1/1
  uncram/3(Out3) -> Mult2/1
  uncram/4(Out4) -> Mult3/1
  uncram1/1(Out1) -> Mult/2
  uncram1/2(Out2) -> Mult1/2
  uncram1/3(Out3) -> Mult2/2
  uncram1/4(Out4) -> Mult3/2
  Mult/1 -> AddSub/1
  Mult1/1 -> AddSub/2
  Mult2/1 -> AddSub1/1
  Mult3/1 -> AddSub1/2
  AddSub/1 -> AddSub2/1
  AddSub1/1 -> AddSub2/2
  AddSub2/1 -> lag/1

== system dbe_xaui_corr/xaui_summer/lag0 ==
  i0 : Inport  OutDataType=sfix(16)  OutScaling=2^0
  q0 : Inport  Port=2  OutDataType=sfix(16)  OutScaling=2^0
  AddSub : xbsIndex_r4/AddSub  mode=Addition  use_carryin=off  use_carryout=off  en=off  latency=2  precision=Full  arith_type=Unsigned  n_bits=16  bin_pt=14  quantization=Truncate  overflow=Wrap  dbl_ovrd=off  use_behavioral_HDL=off  pipelined=off  use_rpm=on  hw_selection=Fabric  block_type=addsub
      settings: block_version=10.1.3
  AddSub1 : xbsIndex_r4/AddSub  mode=Addition  use_carryin=off  use_carryout=off  en=off  latency=2  precision=Full  arith_type=Unsigned  n_bits=16  bin_pt=14  quantization=Truncate  overflow=Wrap  dbl_ovrd=off  use_behavioral_HDL=off  pipelined=off  use_rpm=on  hw_selection=Fabric  block_type=addsub
      settings: block_version=10.1.3
  AddSub2 : xbsIndex_r4/AddSub  mode=Addition  use_carryin=off  use_carryout=off  en=off  latency=2  precision=Full  arith_type=Unsigned  n_bits=16  bin_pt=14  quantization=Truncate  overflow=Wrap  dbl_ovrd=off  use_behavioral_HDL=off  pipelined=off  use_rpm=on  hw_selection=Fabric  block_type=addsub
      settings: block_version=10.1.3
  Delay : xbsIndex_r4/Delay  en=off  latency=1  dbl_ovrd=off  reg_retiming=off  block_type=delay
  Delay1 : xbsIndex_r4/Delay  en=off  latency=1  dbl_ovrd=off  reg_retiming=off  block_type=delay
  Mult{,1..3} (4 alike) : xbsIndex_r4/Mult  precision=Full  arith_type="Signed  (2's comp)"  n_bits=16  bin_pt=14  quantization=Truncate  overflow=Wrap  en=off  latency=5  dbl_ovrd=off  use_behavioral_HDL=on  use_embedded=off  opt=Speed  optimum_pipeline=on  pipeline=on  use_rpm=on  placement_style=Triangular  block_type=mult
      settings: infoedit=Hardware notes: To use the internal pipeline stage of the dedicated multiplier you must select 'Pipeline for maximum performance'.  block_version=10.1.3
  uncram : Subsystem  AncestorBlock=gavrt_library/uncram  mask(uncram){num_slice=4, slice_width=8, bin_pt=7, arith_type=1}
      mask prompts: num_slice "Number of slices"; slice_width "Slice Width"; bin_pt "Output Binary Point"; arith_type "Output Arithmetic Type (0=Unsigned, 1=Signed)"
      mask help: Takes a concatenated input and slices it up into even pieces and reinterprets them as signed fixed point numbers with a given binary point.
      mask init:
      | uncram_init(gcb, ...
      |     'num_slice', num_slice, ...
      |     'slice_width', slice_width, ...
      |     'bin_pt', bin_pt, ...
      |     'arith_type', arith_type);
      settings: AttributesFormatString=Fix_8_7
  uncram1 : Subsystem  AncestorBlock=gavrt_library/uncram  mask(uncram){num_slice=4, slice_width=8, bin_pt=7, arith_type=1}
      mask prompts: num_slice "Number of slices"; slice_width "Slice Width"; bin_pt "Output Binary Point"; arith_type "Output Arithmetic Type (0=Unsigned, 1=Signed)"
      mask help: Takes a concatenated input and slices it up into even pieces and reinterprets them as signed fixed point numbers with a given binary point.
      mask init:
      | uncram_init(gcb, ...
      |     'num_slice', num_slice, ...
      |     'slice_width', slice_width, ...
      |     'bin_pt', bin_pt, ...
      |     'arith_type', arith_type);
      settings: AttributesFormatString=Fix_8_7
  i1 : Outport  OutDataType=sfix(16)  OutScaling=2^0
  q1 : Outport  Port=2  OutDataType=sfix(16)  OutScaling=2^0
  lag : Outport  Port=3  OutDataType=sfix(16)  OutScaling=2^0
  wires:
  i0/1 -> uncram/1(In), Delay/1
  q0/1 -> uncram1/1(In), Delay1/1
  Delay/1 -> i1/1
  Delay1/1 -> q1/1
  uncram/1(Out1) -> Mult/1
  uncram/2(Out2) -> Mult1/1
  uncram/3(Out3) -> Mult2/1
  uncram/4(Out4) -> Mult3/1
  uncram1/1(Out1) -> Mult/2
  uncram1/2(Out2) -> Mult1/2
  uncram1/3(Out3) -> Mult2/2
  uncram1/4(Out4) -> Mult3/2
  Mult/1 -> AddSub/1
  Mult1/1 -> AddSub/2
  Mult2/1 -> AddSub1/1
  Mult3/1 -> AddSub1/2
  AddSub/1 -> AddSub2/1
  AddSub1/1 -> AddSub2/2
  AddSub2/1 -> lag/1

== system dbe_xaui_corr/xaui_summer/lag4 ==
  i0 : Inport  OutDataType=sfix(16)  OutScaling=2^0
  q0 : Inport  Port=2  OutDataType=sfix(16)  OutScaling=2^0
  AddSub : xbsIndex_r4/AddSub  mode=Addition  use_carryin=off  use_carryout=off  en=off  latency=2  precision=Full  arith_type=Unsigned  n_bits=16  bin_pt=14  quantization=Truncate  overflow=Wrap  dbl_ovrd=off  use_behavioral_HDL=off  pipelined=off  use_rpm=on  hw_selection=Fabric  block_type=addsub
      settings: block_version=10.1.3
  AddSub1 : xbsIndex_r4/AddSub  mode=Addition  use_carryin=off  use_carryout=off  en=off  latency=2  precision=Full  arith_type=Unsigned  n_bits=16  bin_pt=14  quantization=Truncate  overflow=Wrap  dbl_ovrd=off  use_behavioral_HDL=off  pipelined=off  use_rpm=on  hw_selection=Fabric  block_type=addsub
      settings: block_version=10.1.3
  AddSub2 : xbsIndex_r4/AddSub  mode=Addition  use_carryin=off  use_carryout=off  en=off  latency=2  precision=Full  arith_type=Unsigned  n_bits=16  bin_pt=14  quantization=Truncate  overflow=Wrap  dbl_ovrd=off  use_behavioral_HDL=off  pipelined=off  use_rpm=on  hw_selection=Fabric  block_type=addsub
      settings: block_version=10.1.3
  Delay : xbsIndex_r4/Delay  en=off  latency=1  dbl_ovrd=off  reg_retiming=off  block_type=delay
  Delay1 : xbsIndex_r4/Delay  en=off  latency=1  dbl_ovrd=off  reg_retiming=off  block_type=delay
  Mult{,1..3} (4 alike) : xbsIndex_r4/Mult  precision=Full  arith_type="Signed  (2's comp)"  n_bits=16  bin_pt=14  quantization=Truncate  overflow=Wrap  en=off  latency=5  dbl_ovrd=off  use_behavioral_HDL=on  use_embedded=off  opt=Speed  optimum_pipeline=on  pipeline=on  use_rpm=on  placement_style=Triangular  block_type=mult
      settings: infoedit=Hardware notes: To use the internal pipeline stage of the dedicated multiplier you must select 'Pipeline for maximum performance'.  block_version=10.1.3
  uncram : Subsystem  AncestorBlock=gavrt_library/uncram  mask(uncram){num_slice=4, slice_width=8, bin_pt=7, arith_type=1}
      mask prompts: num_slice "Number of slices"; slice_width "Slice Width"; bin_pt "Output Binary Point"; arith_type "Output Arithmetic Type (0=Unsigned, 1=Signed)"
      mask help: Takes a concatenated input and slices it up into even pieces and reinterprets them as signed fixed point numbers with a given binary point.
      mask init:
      | uncram_init(gcb, ...
      |     'num_slice', num_slice, ...
      |     'slice_width', slice_width, ...
      |     'bin_pt', bin_pt, ...
      |     'arith_type', arith_type);
      settings: AttributesFormatString=Fix_8_7
  uncram1 : Subsystem  AncestorBlock=gavrt_library/uncram  mask(uncram){num_slice=4, slice_width=8, bin_pt=7, arith_type=1}
      mask prompts: num_slice "Number of slices"; slice_width "Slice Width"; bin_pt "Output Binary Point"; arith_type "Output Arithmetic Type (0=Unsigned, 1=Signed)"
      mask help: Takes a concatenated input and slices it up into even pieces and reinterprets them as signed fixed point numbers with a given binary point.
      mask init:
      | uncram_init(gcb, ...
      |     'num_slice', num_slice, ...
      |     'slice_width', slice_width, ...
      |     'bin_pt', bin_pt, ...
      |     'arith_type', arith_type);
      settings: AttributesFormatString=Fix_8_7
  i1 : Outport  OutDataType=sfix(16)  OutScaling=2^0
  q1 : Outport  Port=2  OutDataType=sfix(16)  OutScaling=2^0
  lag : Outport  Port=3  OutDataType=sfix(16)  OutScaling=2^0
  wires:
  AddSub2/1 -> lag/1
  AddSub1/1 -> AddSub2/2
  AddSub/1 -> AddSub2/1
  Mult3/1 -> AddSub1/2
  Mult2/1 -> AddSub1/1
  Mult1/1 -> AddSub/2
  Mult/1 -> AddSub/1
  uncram1/4(Out4) -> Mult3/2
  uncram1/3(Out3) -> Mult2/2
  uncram1/2(Out2) -> Mult1/2
  uncram1/1(Out1) -> Mult/2
  uncram/4(Out4) -> Mult3/1
  uncram/3(Out3) -> Mult2/1
  uncram/2(Out2) -> Mult1/1
  uncram/1(Out1) -> Mult/1
  Delay1/1 -> q1/1
  Delay/1 -> i1/1
  q0/1 -> Delay1/1, uncram1/1(In)
  i0/1 -> Delay/1, uncram/1(In)

== system dbe_xaui_corr/xaui_summer/lag8 ==
  i0 : Inport  OutDataType=sfix(16)  OutScaling=2^0
  q0 : Inport  Port=2  OutDataType=sfix(16)  OutScaling=2^0
  AddSub : xbsIndex_r4/AddSub  mode=Addition  use_carryin=off  use_carryout=off  en=off  latency=2  precision=Full  arith_type=Unsigned  n_bits=16  bin_pt=14  quantization=Truncate  overflow=Wrap  dbl_ovrd=off  use_behavioral_HDL=off  pipelined=off  use_rpm=on  hw_selection=Fabric  block_type=addsub
      settings: block_version=10.1.3
  AddSub1 : xbsIndex_r4/AddSub  mode=Addition  use_carryin=off  use_carryout=off  en=off  latency=2  precision=Full  arith_type=Unsigned  n_bits=16  bin_pt=14  quantization=Truncate  overflow=Wrap  dbl_ovrd=off  use_behavioral_HDL=off  pipelined=off  use_rpm=on  hw_selection=Fabric  block_type=addsub
      settings: block_version=10.1.3
  AddSub2 : xbsIndex_r4/AddSub  mode=Addition  use_carryin=off  use_carryout=off  en=off  latency=2  precision=Full  arith_type=Unsigned  n_bits=16  bin_pt=14  quantization=Truncate  overflow=Wrap  dbl_ovrd=off  use_behavioral_HDL=off  pipelined=off  use_rpm=on  hw_selection=Fabric  block_type=addsub
      settings: block_version=10.1.3
  Delay : xbsIndex_r4/Delay  en=off  latency=1  dbl_ovrd=off  reg_retiming=off  block_type=delay
  Delay1 : xbsIndex_r4/Delay  en=off  latency=1  dbl_ovrd=off  reg_retiming=off  block_type=delay
  Mult{,1..3} (4 alike) : xbsIndex_r4/Mult  precision=Full  arith_type="Signed  (2's comp)"  n_bits=16  bin_pt=14  quantization=Truncate  overflow=Wrap  en=off  latency=5  dbl_ovrd=off  use_behavioral_HDL=on  use_embedded=off  opt=Speed  optimum_pipeline=on  pipeline=on  use_rpm=on  placement_style=Triangular  block_type=mult
      settings: infoedit=Hardware notes: To use the internal pipeline stage of the dedicated multiplier you must select 'Pipeline for maximum performance'.  block_version=10.1.3
  uncram : Subsystem  AncestorBlock=gavrt_library/uncram  mask(uncram){num_slice=4, slice_width=8, bin_pt=7, arith_type=1}
      mask prompts: num_slice "Number of slices"; slice_width "Slice Width"; bin_pt "Output Binary Point"; arith_type "Output Arithmetic Type (0=Unsigned, 1=Signed)"
      mask help: Takes a concatenated input and slices it up into even pieces and reinterprets them as signed fixed point numbers with a given binary point.
      mask init:
      | uncram_init(gcb, ...
      |     'num_slice', num_slice, ...
      |     'slice_width', slice_width, ...
      |     'bin_pt', bin_pt, ...
      |     'arith_type', arith_type);
      settings: AttributesFormatString=Fix_8_7
  uncram1 : Subsystem  AncestorBlock=gavrt_library/uncram  mask(uncram){num_slice=4, slice_width=8, bin_pt=7, arith_type=1}
      mask prompts: num_slice "Number of slices"; slice_width "Slice Width"; bin_pt "Output Binary Point"; arith_type "Output Arithmetic Type (0=Unsigned, 1=Signed)"
      mask help: Takes a concatenated input and slices it up into even pieces and reinterprets them as signed fixed point numbers with a given binary point.
      mask init:
      | uncram_init(gcb, ...
      |     'num_slice', num_slice, ...
      |     'slice_width', slice_width, ...
      |     'bin_pt', bin_pt, ...
      |     'arith_type', arith_type);
      settings: AttributesFormatString=Fix_8_7
  i1 : Outport  OutDataType=sfix(16)  OutScaling=2^0
  q1 : Outport  Port=2  OutDataType=sfix(16)  OutScaling=2^0
  lag : Outport  Port=3  OutDataType=sfix(16)  OutScaling=2^0
  wires:
  i0/1 -> uncram/1(In), Delay/1
  q0/1 -> uncram1/1(In), Delay1/1
  Delay/1 -> i1/1
  Delay1/1 -> q1/1
  uncram/1(Out1) -> Mult/1
  uncram/2(Out2) -> Mult1/1
  uncram/3(Out3) -> Mult2/1
  uncram/4(Out4) -> Mult3/1
  uncram1/1(Out1) -> Mult/2
  uncram1/2(Out2) -> Mult1/2
  uncram1/3(Out3) -> Mult2/2
  uncram1/4(Out4) -> Mult3/2
  Mult/1 -> AddSub/1
  Mult1/1 -> AddSub/2
  Mult2/1 -> AddSub1/1
  Mult3/1 -> AddSub1/2
  AddSub/1 -> AddSub2/1
  AddSub1/1 -> AddSub2/2
  AddSub2/1 -> lag/1

== system dbe_xaui_corr/xaui_summer/ring_buffer ==
  d : Inport
  delay : Inport  Port=2
  AddSub2 : xbsIndex_r4/AddSub  mode=Subtraction  use_carryin=off  use_carryout=off  en=off  latency=2  precision=User Defined  arith_type=Unsigned  n_bits=4  bin_pt=0  quantization=Truncate  overflow=Wrap  dbl_ovrd=off  use_behavioral_HDL=off  pipelined=on  use_rpm=on  hw_selection=Fabric  block_type=addsub
      settings: block_version=10.1.3
  Constant : xbsIndex_r4/Constant  arith_type=Boolean  const=1  n_bits=16  bin_pt=14  explicit_period=on  period=1  equ=P=C  opselect=C  inp2=PCIN>>17  opr=+  inp1=P  carry=CIN  dbl_ovrd=off  block_type=constant
  Constant1 : xbsIndex_r4/Constant  arith_type=Boolean  const=0  n_bits=16  bin_pt=14  explicit_period=on  period=1  equ=P=C  opselect=C  inp2=PCIN>>17  opr=+  inp1=P  carry=CIN  dbl_ovrd=off  block_type=constant
  Constant3 : xbsIndex_r4/Constant  arith_type=Unsigned  const=0  n_bits=32  bin_pt=0  explicit_period=on  period=1  equ=P=C  opselect=C  inp2=PCIN>>17  opr=+  inp1=P  carry=CIN  dbl_ovrd=off  block_type=constant
  Counter : xbsIndex_r4/Counter  cnt_type=Free Running  cnt_to=Inf  operation=Up  start_count=0  cnt_by_val=1  arith_type=Unsigned  n_bits=4  bin_pt=0  load_pin=off  rst=off  en=off  explicit_period=on  period=1  dbl_ovrd=off  use_behavioral_HDL=off  use_rpm=off  implementation=Fabric  block_type=counter
  Delay5 : xbsIndex_r4/Delay  en=off  latency=2  dbl_ovrd=off  reg_retiming=on  block_type=delay
  dpr16 : xbsIndex_r4/Dual Port RAM  depth=16  initVector=zeros(1,16)  distributed_mem=Block RAM  init_a=0  init_b=0  rst_a=off  rst_b=off  en_a=off  en_b=off  latency=1  write_mode_A=Read After Write  write_mode_B=Read After Write  dbl_ovrd=off  optimize=Speed  use_rpm=on  block_type=dpram
      settings: block_version=10.1.3
  q0 : Outport
  qdel : Outport  Port=2
  wires:
  Delay5/1 -> dpr16/1
  Counter/1 -> Delay5/1, AddSub2/1
  AddSub2/1 -> dpr16/4
  Constant/1 -> dpr16/3
  Constant1/1 -> dpr16/6
  Constant3/1 -> dpr16/5
  d/1 -> dpr16/2
  dpr16/1 -> q0/1
  delay/1 -> AddSub2/2
  dpr16/2 -> qdel/1
